simulink model "transform"  (Simulink 7.5)
settings: Solver=ode45  StartTime=0.0  StopTime=10.0  RelTol=1e-3
settings Model: Creator=knightofaccess  LastModifiedBy=knightofaccess

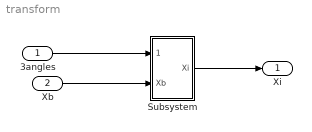
== system transform ==
  3angles : Inport  OutDataType=sfix(16)  OutScaling=2^0
  Xb : Inport  Port=2  OutDataType=sfix(16)  OutScaling=2^0
  Subsystem : Subsystem
  Xi : Outport  OutDataType=fixdt(1, 16)  OutScaling=2^0
  wires:
  3angles/1 -> Subsystem/1(3angles)
  Xb/1 -> Subsystem/2(Xb)
  Subsystem/1(Xi) -> Xi/1

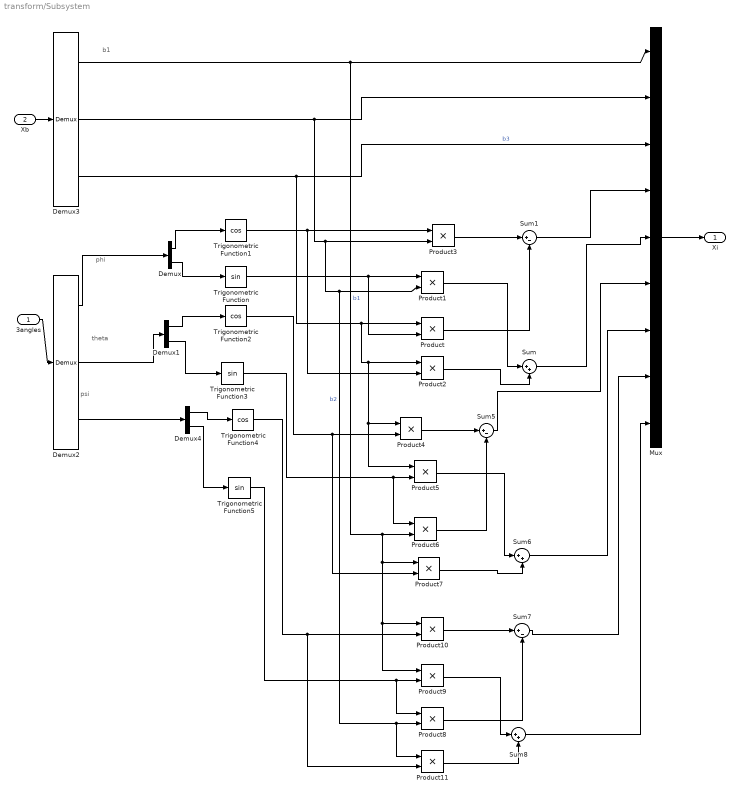
== system transform/Subsystem ==
  note: phi
  note: theta
  note: psi
  note: b1
  3angles : Inport  OutDataType=sfix(16)  OutScaling=2^0
  Xb : Inport  Port=2  OutDataType=sfix(16)  OutScaling=2^0
  Demux : Demux  Outputs=2
  Demux1 : Demux  Outputs=2
  Demux2 : Demux  Outputs=3
  Demux3 : Demux  Outputs=3
  Demux4 : Demux  Outputs=2
  Mux : Mux  Inputs=9
  Product{,1..11} (12 alike) : Product  OutDataType=fixdt(1, 16)  OutScaling=2^0  RndMeth=Zero
  Sum : Sum  Inputs=|++  OutDataType=fixdt(1, 16)  OutScaling=2^0
  Sum1 : Sum  Inputs=|+-  OutDataType=fixdt(1, 16)  OutScaling=2^0
  Sum5 : Sum  Inputs=|+-  OutDataType=fixdt(1, 16)  OutScaling=2^0
  Sum6 : Sum  Inputs=|++  OutDataType=fixdt(1, 16)  OutScaling=2^0
  Sum7 : Sum  Inputs=|+-  OutDataType=fixdt(1, 16)  OutScaling=2^0
  Sum8 : Sum  Inputs=|++  OutDataType=fixdt(1, 16)  OutScaling=2^0
  Trigonometric Function : Trigonometry
  Trigonometric Function1 : Trigonometry  Operator=cos
  Trigonometric Function2 : Trigonometry  Operator=cos
  Trigonometric Function3 : Trigonometry
  Trigonometric Function4 : Trigonometry  Operator=cos
  Trigonometric Function5 : Trigonometry
  Xi : Outport  OutDataType=fixdt(1, 16)  OutScaling=2^0
  wires:
  Demux2/1 -> Demux/1
  Demux/1 -> Trigonometric Function1/1
  Demux/2 -> Trigonometric Function/1
  Demux2/2 -> Demux1/1
  Demux1/1 -> Trigonometric Function2/1
  Demux1/2 -> Trigonometric Function3/1
  3angles/1 -> Demux2/1
  Xb/1 -> Demux3/1
  Demux3/1 -> Mux/1, Product6/2, Product7/1, Product10/1, Product9/1  "b1"
  Demux3/2 -> Mux/2, Product3/2, Product1/2, Product8/2, Product11/1  "b2"
  Demux3/3 -> Mux/3, Product/1, Product2/1, Product4/1, Product5/1  "b3"
  Trigonometric Function1/1 -> Product3/1, Product2/2
  Trigonometric Function/1 -> Product1/1, Product/2
  Product3/1 -> Sum1/1
  Product/1 -> Sum1/2
  Sum1/1 -> Mux/4
  Product1/1 -> Sum/1
  Product2/1 -> Sum/2
  Sum/1 -> Mux/5
  Trigonometric Function2/1 -> Product4/2, Product7/2
  Trigonometric Function3/1 -> Product5/2, Product6/1
  Product4/1 -> Sum5/1
  Product6/1 -> Sum5/2
  Product5/1 -> Sum6/1
  Product7/1 -> Sum6/2
  Sum5/1 -> Mux/6
  Sum6/1 -> Mux/7
  Trigonometric Function4/1 -> Product10/2, Product11/2
  Demux2/3 -> Demux4/1
  Demux4/1 -> Trigonometric Function4/1
  Demux4/2 -> Trigonometric Function5/1
  Trigonometric Function5/1 -> Product9/2, Product8/1
  Product10/1 -> Sum7/1
  Product8/1 -> Sum7/2
  Product9/1 -> Sum8/1
  Product11/1 -> Sum8/2
  Sum7/1 -> Mux/8
  Sum8/1 -> Mux/9
  Mux/1 -> Xi/1
